simulink model "EdgeDetectionPicture"  (Simulink 6.5)
settings: Solver=ode45  StartTime=0.0  StopTime=0  RelTol=1e-3
undefined symbols (not defined in the file or in its folder): jet, Rec, SDTV
libraries: vipsnks x2, vipconversions x1, vipanalysis x1, vipsrcs x1
settings Model: Creator=greith  LastModifiedBy=jacobf

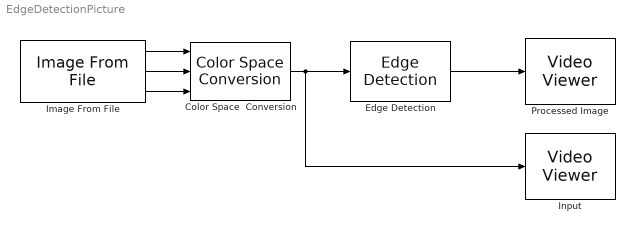
== system EdgeDetectionPicture ==
  Color Space  Conversion : vipconversions/Color Space  Conversion  conversion=R'G'B' to intensity  wp_str=D65  rec=Rec. 601 (SDTV)  sys=1125/60/2:1
  Edge Detection : vipanalysis/Edge Detection  DialogController=vipDDGCreate  DialogControllerArgs=DataTag0  method=Sobel  outputType=Binary image  userDefinedThreshold=off  thresholdSource=Input port  threshold=20  thresholdTuning=1  edgeThinning=off  threshold_canny=[0.25 0.60]  autoPercent=70  sigma=1  prodOutputMode=Binary point scaling  prodOutputWordLength=32  prodOutputFracLength=8  roundingMode=Floor  overflowMode=off
  Image From File : vipsrcs/Image From File  DialogController=vipDDGCreate  DialogControllerArgs=DataTag1  SystemSampleTime=-1  FileName=TMW2.jpg  Ts=inf  ImageDataType=Inherit from input image  Signed=on  WordLength=16  sdImageDataType=uint(8)  FractionLengthMode=User-defined  FractionLength=15  OutPortLabels=R|G|B
  Input : vipsnks/Video Viewer  inputType=Intensity  useColorMap=off  colormapValue=jet(256);  specRange=off  minInputVal=0  maxInputVal=255  FigPos=[622 594 676 470]  AxisZoom=on  trueSizedOnce=on
  Processed Image : vipsnks/Video Viewer  inputType=Intensity  useColorMap=off  colormapValue=jet(256);  specRange=off  minInputVal=0  maxInputVal=255  FigPos=[622 594 676 470]  AxisZoom=on  trueSizedOnce=on
  wires:
  Image From File/1 -> Color Space  Conversion/1
  Image From File/2 -> Color Space  Conversion/2
  Image From File/3 -> Color Space  Conversion/3
  Color Space  Conversion/1 -> Edge Detection/1, Input/1
  Edge Detection/1 -> Processed Image/1
